simulink model "mrefrobotarm_previous_y_previous_u_previous_ref_cex_3"  (R2018b)
settings: Solver=FixedStepAuto  StartTime=0.0  StopTime=20  RelTol=1e-3  AbsTol=1e-6
undefined symbols (not defined in the file or in its folder): cc, options
libraries: neural x396, simulink x2
(part 9 of 15)

== system mrefrobotarm_previous_y_previous_u_previous_ref_cex_3/cex_m3_adapt/Layer 3/Delays 1 ==
  "p{3}" : Inport  PortDimensions=30
      mask Display: e = 0.06;c1 = [120 230 180]/255;c2 = ([120 230 180]+0)/(256+128);c3 = ([120 230 180]+128)/(256+128);patch([0 1 1 0],[0 0 1 1],c1);patch([0 1 1 1-e 1-e 0+e],[0 0 1 1-e 0+e 0+e],c2);patch([0 0 1 1-e 0+e 0+e],[0 1 1 1-e 1-e 0+e],c3);plot([0 1 1 0 0],[0 0 1 1 0]);
  mux : Mux  Inputs=1
      mask Display: e = 0.06;c1 = [120 150 230]/255;c2 = ([120 150 230]+0)/383;c3 = ([120 150 230]+128)/383;patch([0 1 1 0],[0 0 1 1],c1);patch([0 1 1 1-e 1-e 0+e],[0 0 1 1-e 0+e 0+e],c2);patch([0 0 1 1-e 0+e 0+e],[0 1 1 1-e 1-e 0+e],c3);plot([0 1 1 0 0],[0 0 1 1 0]);disp('Mux')
  "pd{3,2}" : Outport
      mask Display: e = 0.06;c1 = [120 230 180]/255;c2 = ([120 230 180]+0)/(256+128);c3 = ([120 230 180]+128)/(256+128);patch([0 1 1 0],[0 0 1 1],c1);patch([0 1 1 1-e 1-e 0+e],[0 0 1 1-e 0+e 0+e],c2);patch([0 0 1 1-e 0+e 0+e],[0 1 1 1-e 1-e 0+e],c3);plot([0 1 1 0 0],[0 0 1 1 0]);
  wires:
  "p{3}"/1 -> mux/1
  mux/1 -> "pd{3,2}"/1

== system mrefrobotarm_previous_y_previous_u_previous_ref_cex_3/cex_m3_adapt/Layer 3/LW{3,2} ==
  "ad{3,2}" : Inport  PortDimensions=30
      mask Display: e = 0.06;c1 = [120 230 180]/255;c2 = ([120 230 180]+0)/(256+128);c3 = ([120 230 180]+128)/(256+128);patch([0 1 1 0],[0 0 1 1],c1);patch([0 1 1 1-e 1-e 0+e],[0 0 1 1-e 0+e 0+e],c2);patch([0 0 1 1-e 0+e 0+e],[0 1 1 1-e 1-e 0+e],c3);plot([0 1 1 0 0],[0 0 1 1 0]);
  "IW{3,2}(1,:)'" : Constant  Value=[-0.0550595154242625728358007108909077942371368408203125;-0.3289027625891562944815404989640228450298309326171875;0.415393748344756452706150184894795529544353485107421875;-0.2282636721929082457283044504947611130774021148681640625;0.1668741853640021977067675607031560502946376800537109375;-0.287669874496869149016475830649142153561115264892578125;-0.3212911955461403845646373156341724097728729248046875;0.12071215019926258282811915023557958193123340606689453125;-0.0146013532017180598654437773120662313885986804962158203125;0.50163897067026586018556599810835905373096466064453125;0.35771292541943811027493893561768345534801483154296875;-0.00629606603251300737944529117839920218102633953094482421875;-0.04508272836454159382402195888062124140560626983642578125;0.00996937137599121676878599629390009795315563678741455078125;0.285260980440774691846428368080523796379566192626953125;0.2491459745752436505394911137045710347592830657958984375;-0.183824283017604284129475900044781155884265899658203125;0.45987709705359447465156108592054806649684906005859375;0.03695776745205560376295039759497740305960178375244140625;0.038818132468089842912473130809303256683051586151123046875;0.32020077507497279878379004003363661468029022216796875;-0.02219398795991646411440711972318240441381931304931640625;0.176419324787934705955905201335554011166095733642578125;-0.369064045925398043213050414124154485762119293212890625;-0.0296495007456062768802507179088934208266437053680419921875;-0.03653538424870143852540849138677003793418407440185546875;0.278071205950087219083144418618758209049701690673828125;0.5598987685029681582449256893596611917018890380859375;-0.2178278744586039927799703264099662192165851593017578125;0.406415787608162049071580668169190175831317901611328125]
      mask Display: e = 0.06;c1 = [120 150 230]/255;c2 = ([120 150 230]+0)/383;c3 = ([120 150 230]+128)/383;patch([0 1 1 0],[0 0 1 1],c1);patch([0 1 1 1-e 1-e 0+e],[0 0 1 1-e 0+e 0+e],c2);patch([0 0 1 1-e 0+e 0+e],[0 1 1 1-e 1-e 0+e],c3);plot([0 1 1 0 0],[0 0 1 1 0]);disp('weights');
  Mux : Mux  Inputs=1
      mask Display: e = 0.06;c1 = [120 150 230]/255;c2 = ([120 150 230]+0)/383;c3 = ([120 150 230]+128)/383;patch([0 1 1 0],[0 0 1 1],c1);patch([0 1 1 1-e 1-e 0+e],[0 0 1 1-e 0+e 0+e],c2);patch([0 0 1 1-e 0+e 0+e],[0 1 1 1-e 1-e 0+e],c3);plot([0 1 1 0 0],[0 0 1 1 0]);disp('Mux');
  dotprod1 : neural/Weight Functions/dotprod
  "lz{3,2}" : Outport
      mask Display: e = 0.06;c1 = [120 230 180]/255;c2 = ([120 230 180]+0)/(256+128);c3 = ([120 230 180]+128)/(256+128);patch([0 1 1 0],[0 0 1 1],c1);patch([0 1 1 1-e 1-e 0+e],[0 0 1 1-e 0+e 0+e],c2);patch([0 0 1 1-e 0+e 0+e],[0 1 1 1-e 1-e 0+e],c3);plot([0 1 1 0 0],[0 0 1 1 0]);
  wires:
  "IW{3,2}(1,:)'"/1 -> dotprod1/1
  "ad{3,2}"/1 -> dotprod1/2
  dotprod1/1 -> Mux/1
  Mux/1 -> "lz{3,2}"/1

== system mrefrobotarm_previous_y_previous_u_previous_ref_cex_3/cex_m4_10_cl/Layer 1/Delays 1 ==
  "p{1}" : Inport  PortDimensions=10
      mask Display: e = 0.06;c1 = [120 230 180]/255;c2 = ([120 230 180]+0)/(256+128);c3 = ([120 230 180]+128)/(256+128);patch([0 1 1 0],[0 0 1 1],c1);patch([0 1 1 1-e 1-e 0+e],[0 0 1 1-e 0+e 0+e],c2);patch([0 0 1 1-e 0+e 0+e],[0 1 1 1-e 1-e 0+e],c3);plot([0 1 1 0 0],[0 0 1 1 0]);
  mux : Mux  Inputs=1
      mask Display: e = 0.06;c1 = [120 150 230]/255;c2 = ([120 150 230]+0)/383;c3 = ([120 150 230]+128)/383;patch([0 1 1 0],[0 0 1 1],c1);patch([0 1 1 1-e 1-e 0+e],[0 0 1 1-e 0+e 0+e],c2);patch([0 0 1 1-e 0+e 0+e],[0 1 1 1-e 1-e 0+e],c3);plot([0 1 1 0 0],[0 0 1 1 0]);disp('Mux')
  "pd{1,1}" : Outport
      mask Display: e = 0.06;c1 = [120 230 180]/255;c2 = ([120 230 180]+0)/(256+128);c3 = ([120 230 180]+128)/(256+128);patch([0 1 1 0],[0 0 1 1],c1);patch([0 1 1 1-e 1-e 0+e],[0 0 1 1-e 0+e 0+e],c2);patch([0 0 1 1-e 0+e 0+e],[0 1 1 1-e 1-e 0+e],c3);plot([0 1 1 0 0],[0 0 1 1 0]);
  wires:
  "p{1}"/1 -> mux/1
  mux/1 -> "pd{1,1}"/1

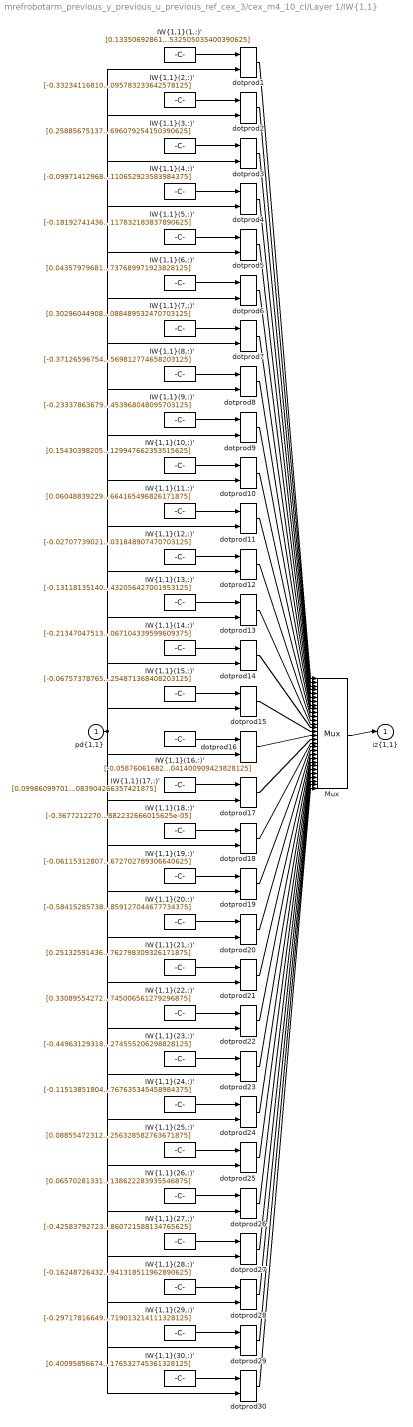
== system mrefrobotarm_previous_y_previous_u_previous_ref_cex_3/cex_m4_10_cl/Layer 1/IW{1,1} ==
  "pd{1,1}" : Inport  PortDimensions=10
      mask Display: e = 0.06;c1 = [120 230 180]/255;c2 = ([120 230 180]+0)/(256+128);c3 = ([120 230 180]+128)/(256+128);patch([0 1 1 0],[0 0 1 1],c1);patch([0 1 1 1-e 1-e 0+e],[0 0 1 1-e 0+e 0+e],c2);patch([0 0 1 1-e 0+e 0+e],[0 1 1 1-e 1-e 0+e],c3);plot([0 1 1 0 0],[0 0 1 1 0]);
  "IW{1,1}(1,:)'" : Constant  Value=[0.1335069286146624290001483359446865506470203399658203125;-0.04119881948015781392147260930869379080832004547119140625;-0.04923129418669790202667257972279912792146205902099609375;-0.11541957449396934853869112203028635121881961822509765625;-0.1293441358240161320747318995927344076335430145263671875;-0.044315180700797374147015261769411154091358184814453125;-0.30838951010690951459736197648453526198863983154296875;0.10507902740775072747414498053331044502556324005126953125;-0.2124968740055101223962452650084742344915866851806640625;0.2253827290816003137141620982220047153532505035400390625]
      mask Display: e = 0.06;c1 = [120 150 230]/255;c2 = ([120 150 230]+0)/383;c3 = ([120 150 230]+128)/383;patch([0 1 1 0],[0 0 1 1],c1);patch([0 1 1 1-e 1-e 0+e],[0 0 1 1-e 0+e 0+e],c2);patch([0 0 1 1-e 0+e 0+e],[0 1 1 1-e 1-e 0+e],c3);plot([0 1 1 0 0],[0 0 1 1 0]);disp('Weights');
  "IW{1,1}(10,:)'" : Constant  Value=[0.1543039820570023257229053115224814973771572113037109375;0.44163458230561747352993506865459494292736053466796875;-0.157209668123826862284886374254710972309112548828125;0.1729117581733836950252936048855190165340900421142578125;0.43717240672936885648169891283032484352588653564453125;-0.185011277685246167123978011659346520900726318359375;0.243474939005600299335441150105907581746578216552734375;-0.0010861071418907385262297982109203076106496155261993408203125;0.1532198832903562124574392555587110109627246856689453125;-0.06418866992842099661320531822639168240129947662353515625]
      mask Display: e = 0.06;c1 = [120 150 230]/255;c2 = ([120 150 230]+0)/383;c3 = ([120 150 230]+128)/383;patch([0 1 1 0],[0 0 1 1],c1);patch([0 1 1 1-e 1-e 0+e],[0 0 1 1-e 0+e 0+e],c2);patch([0 0 1 1-e 0+e 0+e],[0 1 1 1-e 1-e 0+e],c3);plot([0 1 1 0 0],[0 0 1 1 0]);disp('Weights');
  "IW{1,1}(11,:)'" : Constant  Value=[0.0604883922918798833112674628864624537527561187744140625;-0.12877197402082496413555645631277002394199371337890625;-0.0183281447432761500360154371946919127367436885833740234375;-0.17418874047358390289019780539092607796192169189453125;0.0248699482724969618552268713074226980097591876983642578125;0.262836414092244174955936841797665692865848541259765625;-0.134245057446654325605805979648721404373645782470703125;0.1889774580328676123475162285103579051792621612548828125;-0.0915680536010251844292184841833659447729587554931640625;0.074272479267489088794462759324233047664165496826171875]
      mask Display: e = 0.06;c1 = [120 150 230]/255;c2 = ([120 150 230]+0)/383;c3 = ([120 150 230]+128)/383;patch([0 1 1 0],[0 0 1 1],c1);patch([0 1 1 1-e 1-e 0+e],[0 0 1 1-e 0+e 0+e],c2);patch([0 0 1 1-e 0+e 0+e],[0 1 1 1-e 1-e 0+e],c3);plot([0 1 1 0 0],[0 0 1 1 0]);disp('Weights');
  "IW{1,1}(12,:)'" : Constant  Value=[-0.0270773902183627200590532169144353247247636318206787109375;-0.3935532540680071189598265846143476665019989013671875;0.1544558044375887728705265544704161584377288818359375;0.1135619620646874938785231279325671494007110595703125;-0.06923700442986756298235917483907542191445827484130859375;0.023714916382562567509495465856161899864673614501953125;-0.2434424848174343569695565747679211199283599853515625;-0.1940819242046150361336032119652372784912586212158203125;0.1772986216597098041436453286223695613443851470947265625;-0.1902225870534570983938493782261502929031848907470703125]
      mask Display: e = 0.06;c1 = [120 150 230]/255;c2 = ([120 150 230]+0)/383;c3 = ([120 150 230]+128)/383;patch([0 1 1 0],[0 0 1 1],c1);patch([0 1 1 1-e 1-e 0+e],[0 0 1 1-e 0+e 0+e],c2);patch([0 0 1 1-e 0+e 0+e],[0 1 1 1-e 1-e 0+e],c3);plot([0 1 1 0 0],[0 0 1 1 0]);disp('Weights');
  "IW{1,1}(13,:)'" : Constant  Value=[-0.131181351403738821748135023881332017481327056884765625;0.1362970166403306981894871796612278558313846588134765625;-0.0631587600902037415995238234245334751904010772705078125;0.1979319007788440110129357663026894442737102508544921875;-0.14152574162728093210006363733555190265178680419921875;0.00842057206973761095125663445060126832686364650726318359375;0.0918117915633907266670377111950074322521686553955078125;-0.15022518079095015242074850903009064495563507080078125;-0.199192862120646629886522305241669528186321258544921875;0.292466314204549437949509638201561756432056427001953125]
      mask Display: e = 0.06;c1 = [120 150 230]/255;c2 = ([120 150 230]+0)/383;c3 = ([120 150 230]+128)/383;patch([0 1 1 0],[0 0 1 1],c1);patch([0 1 1 1-e 1-e 0+e],[0 0 1 1-e 0+e 0+e],c2);patch([0 0 1 1-e 0+e 0+e],[0 1 1 1-e 1-e 0+e],c3);plot([0 1 1 0 0],[0 0 1 1 0]);disp('Weights');
  "IW{1,1}(14,:)'" : Constant  Value=[-0.21347047513201877766420011539594270288944244384765625;0.016920838378240217469983264209076878614723682403564453125;0.26282359254795928382719694127445109188556671142578125;-0.038626445771948618446156586969664203934371471405029296875;0.01267614658551742719272414916531488415785133838653564453125;0.243713695853148115677555551883415319025516510009765625;0.232007573027820435118684372355346567928791046142578125;0.292359098771159120477847181973629631102085113525390625;-0.1367485882737829727684442104873596690595149993896484375;0.0747256641880101601937980149159557186067104339599609375]
      mask Display: e = 0.06;c1 = [120 150 230]/255;c2 = ([120 150 230]+0)/383;c3 = ([120 150 230]+128)/383;patch([0 1 1 0],[0 0 1 1],c1);patch([0 1 1 1-e 1-e 0+e],[0 0 1 1-e 0+e 0+e],c2);patch([0 0 1 1-e 0+e 0+e],[0 1 1 1-e 1-e 0+e],c3);plot([0 1 1 0 0],[0 0 1 1 0]);disp('Weights');
  "IW{1,1}(15,:)'" : Constant  Value=[-0.067573787655347938851946310023777186870574951171875;-0.295392823875792964738451473749591968953609466552734375;-0.0168225079369467185597120106876900536008179187774658203125;-0.297859471899082295376359752481221221387386322021484375;-0.28145973576240546076832060862216167151927947998046875;-0.2100793210813916844781346071613370440900325775146484375;0.0167045522183084625689186708541456027887761592864990234375;-0.243409163141346918113328001709305681288242340087890625;0.1817946730395441912175868992562755011022090911865234375;-0.018388171280658067996416349387800437398254871368408203125]
      mask Display: e = 0.06;c1 = [120 150 230]/255;c2 = ([120 150 230]+0)/383;c3 = ([120 150 230]+128)/383;patch([0 1 1 0],[0 0 1 1],c1);patch([0 1 1 1-e 1-e 0+e],[0 0 1 1-e 0+e 0+e],c2);patch([0 0 1 1-e 0+e 0+e],[0 1 1 1-e 1-e 0+e],c3);plot([0 1 1 0 0],[0 0 1 1 0]);disp('Weights');
  "IW{1,1}(16,:)'" : Constant  Value=[-0.05876061682829540611106011738229426555335521697998046875;0.360436775341689052964966322178952395915985107421875;0.289705563067306937075073847154271788895130157470703125;0.12081195104620233438108556356382905505597591400146484375;-0.1033261310861984527686985302352695725858211517333984375;0.2466138189248444356760359141844674013555049896240234375;0.21455052857311296410358636421733535826206207275390625;-0.08664495004047449711048756171294371597468852996826171875;0.1862050765935379381676995080852066166698932647705078125;-0.052106136261183162716736916308946092613041400909423828125]
      mask Display: e = 0.06;c1 = [120 150 230]/255;c2 = ([120 150 230]+0)/383;c3 = ([120 150 230]+128)/383;patch([0 1 1 0],[0 0 1 1],c1);patch([0 1 1 1-e 1-e 0+e],[0 0 1 1-e 0+e 0+e],c2);patch([0 0 1 1-e 0+e 0+e],[0 1 1 1-e 1-e 0+e],c3);plot([0 1 1 0 0],[0 0 1 1 0]);disp('Weights');
  "IW{1,1}(17,:)'" : Constant  Value=[0.09986099701258464855779806157443090341985225677490234375;-0.06888901320057617960745943719302886165678501129150390625;-0.09200685624381586824593881601686007343232631683349609375;-0.1891588439145970301780153022264130413532257080078125;0.113842455384469520840440281972405500710010528564453125;0.032373501675791165055340314893328468315303325653076171875;0.0486132218901944579414475811063311994075775146484375;-0.2115118545103817082608799182708025909960269927978515625;-0.2031023047480521592778046624516719020903110504150390625;-0.329202134434376680882650134662981145083904266357421875]
      mask Display: e = 0.06;c1 = [120 150 230]/255;c2 = ([120 150 230]+0)/383;c3 = ([120 150 230]+128)/383;patch([0 1 1 0],[0 0 1 1],c1);patch([0 1 1 1-e 1-e 0+e],[0 0 1 1-e 0+e 0+e],c2);patch([0 0 1 1-e 0+e 0+e],[0 1 1 1-e 1-e 0+e],c3);plot([0 1 1 0 0],[0 0 1 1 0]);disp('Weights');
  "IW{1,1}(18,:)'" : Constant  Value=[-0.3677212270391405635194814749411307275295257568359375;0.05148060778210650223485345122753642499446868896484375;-0.093255280771188997501752737662172876298427581787109375;0.06565608607994800893781217610012390650808811187744140625;-0.225727788425362951851838033690000884234905242919921875;0.09605090868460068598277956652964348904788494110107421875;0.033920970624489343858698475742130540311336517333984375;-0.26114541967138749090082683323998935520648956298828125;0.257344020629603875693902637067367322742938995361328125;-8.736879148670711504875985298212981433607637882232666015625e-05]
      mask Display: e = 0.06;c1 = [120 150 230]/255;c2 = ([120 150 230]+0)/383;c3 = ([120 150 230]+128)/383;patch([0 1 1 0],[0 0 1 1],c1);patch([0 1 1 1-e 1-e 0+e],[0 0 1 1-e 0+e 0+e],c2);patch([0 0 1 1-e 0+e 0+e],[0 1 1 1-e 1-e 0+e],c3);plot([0 1 1 0 0],[0 0 1 1 0]);disp('Weights');
  "IW{1,1}(19,:)'" : Constant  Value=[-0.061153128073666941644237482478274614550173282623291015625;-0.150089827624216354262642880712519399821758270263671875;0.08671999110216542516749171909395954571664333343505859375;-0.0628523003683129355412262384561472572386264801025390625;0.2452322268404465710478490336754475720226764678955078125;-0.10162074530770455471628821442209300585091114044189453125;0.334201538400112851956436088585178367793560028076171875;0.009410034126397896769855577758789877407252788543701171875;-0.1646375700629976457367575903845136053860187530517578125;-0.11189823007734533977242108448990620672702789306640625]
      mask Display: e = 0.06;c1 = [120 150 230]/255;c2 = ([120 150 230]+0)/383;c3 = ([120 150 230]+128)/383;patch([0 1 1 0],[0 0 1 1],c1);patch([0 1 1 1-e 1-e 0+e],[0 0 1 1-e 0+e 0+e],c2);patch([0 0 1 1-e 0+e 0+e],[0 1 1 1-e 1-e 0+e],c3);plot([0 1 1 0 0],[0 0 1 1 0]);disp('Weights');
  "IW{1,1}(2,:)'" : Constant  Value=[-0.3323411681062318212553918783669359982013702392578125;-0.154673593400318776236446183247608132660388946533203125;0.1653441009670726102864790618696133606135845184326171875;0.08240688446507839215460222703768522478640079498291015625;0.286432838047223470301361203382839448750019073486328125;-0.022122764349317834697838947022319189272820949554443359375;-0.00766446205364790418557152662515363772399723529815673828125;-0.1367725418678419069262730545233353041112422943115234375;-0.250579344929661218532856992169399745762348175048828125;0.053861527883418525153302880426053889095783233642578125]
      mask Display: e = 0.06;c1 = [120 150 230]/255;c2 = ([120 150 230]+0)/383;c3 = ([120 150 230]+128)/383;patch([0 1 1 0],[0 0 1 1],c1);patch([0 1 1 1-e 1-e 0+e],[0 0 1 1-e 0+e 0+e],c2);patch([0 0 1 1-e 0+e 0+e],[0 1 1 1-e 1-e 0+e],c3);plot([0 1 1 0 0],[0 0 1 1 0]);disp('Weights');
  "IW{1,1}(20,:)'" : Constant  Value=[-0.58415285738136812909715445130132138729095458984375;0.53930070079611847067013741252594627439975738525390625;-0.197661936388412673437642297358252108097076416015625;-0.1690839785960029095779333374593988992273807525634765625;-0.00690086496233999029115135925849244813434779644012451171875;-0.419685250641533780235903350330772809684276580810546875;-0.09872138899374226228555784246054827235639095306396484375;-0.1627977525170371808638236643673735670745372772216796875;-0.318146809739166924746456288630724884569644927978515625;-0.130148046874022094154810247346176765859127044677734375]
      mask Display: e = 0.06;c1 = [120 150 230]/255;c2 = ([120 150 230]+0)/383;c3 = ([120 150 230]+128)/383;patch([0 1 1 0],[0 0 1 1],c1);patch([0 1 1 1-e 1-e 0+e],[0 0 1 1-e 0+e 0+e],c2);patch([0 0 1 1-e 0+e 0+e],[0 1 1 1-e 1-e 0+e],c3);plot([0 1 1 0 0],[0 0 1 1 0]);disp('Weights');
  "IW{1,1}(21,:)'" : Constant  Value=[0.251325914363370983561907223702291958034038543701171875;0.179997632412586094918793833130621351301670074462890625;0.2489681945741413215955617488361895084381103515625;-0.10037777365444662536209108338880469091236591339111328125;-0.152924777124262278871213993625133298337459564208984375;0.282206938701535847702217552068759687244892120361328125;-0.161723546504821624747449959613732062280178070068359375;0.12769054485279285326981835169135592877864837646484375;0.2150941775257640131702174812744488008320331573486328125;-0.0186245132798998624945596702673356048762798309326171875]
      mask Display: e = 0.06;c1 = [120 150 230]/255;c2 = ([120 150 230]+0)/383;c3 = ([120 150 230]+128)/383;patch([0 1 1 0],[0 0 1 1],c1);patch([0 1 1 1-e 1-e 0+e],[0 0 1 1-e 0+e 0+e],c2);patch([0 0 1 1-e 0+e 0+e],[0 1 1 1-e 1-e 0+e],c3);plot([0 1 1 0 0],[0 0 1 1 0]);disp('Weights');
  "IW{1,1}(22,:)'" : Constant  Value=[0.33089554272644416954562984756194055080413818359375;-0.1924353896389504325892261249464354477822780609130859375;-0.2267754942334463674757927265090984292328357696533203125;-0.0934872108709188243125254302867688238620758056640625;-0.054699933021623577122927173377320286817848682403564453125;0.035072794239530420690176271136806462891399860382080078125;0.26562875685814424375763564967201091349124908447265625;-0.0791922808190812232975730466932873241603374481201171875;0.0521094046242211172970115740099572576582431793212890625;0.339894278826450235708733771389233879745006561279296875]
      mask Display: e = 0.06;c1 = [120 150 230]/255;c2 = ([120 150 230]+0)/383;c3 = ([120 150 230]+128)/383;patch([0 1 1 0],[0 0 1 1],c1);patch([0 1 1 1-e 1-e 0+e],[0 0 1 1-e 0+e 0+e],c2);patch([0 0 1 1-e 0+e 0+e],[0 1 1 1-e 1-e 0+e],c3);plot([0 1 1 0 0],[0 0 1 1 0]);disp('Weights');
  "IW{1,1}(23,:)'" : Constant  Value=[-0.449631293180019764310628715975326485931873321533203125;-0.07520771148848910681028456792773795314133167266845703125;0.201995553128253402253022841250640340149402618408203125;0.0879938416974312687113268793837050907313823699951171875;0.276521095050688614502831796926329843699932098388671875;-0.00327530247935484651600201999599448754452168941497802734375;-0.08464502029784491676789315306450589559972286224365234375;-0.06796671234375029069241236356901936233043670654296875;0.252160726035627058561061630825861357152462005615234375;-0.23821476079948400439434408326633274555206298828125]
      mask Display: e = 0.06;c1 = [120 150 230]/255;c2 = ([120 150 230]+0)/383;c3 = ([120 150 230]+128)/383;patch([0 1 1 0],[0 0 1 1],c1);patch([0 1 1 1-e 1-e 0+e],[0 0 1 1-e 0+e 0+e],c2);patch([0 0 1 1-e 0+e 0+e],[0 1 1 1-e 1-e 0+e],c3);plot([0 1 1 0 0],[0 0 1 1 0]);disp('Weights');
  "IW{1,1}(24,:)'" : Constant  Value=[-0.11513851804525521149713540580705739557743072509765625;0.2108759995406740139767265418413444422185420989990234375;-0.150452927119801349586936112245894037187099456787109375;0.313006723398378483569359786997665651142597198486328125;0.1500465352567468546585160993345198221504688262939453125;0.257667967348261306437251505485619418323040008544921875;0.12369309318535488817492051794033613987267017364501953125;0.07888033237337994940663321585816447623074054718017578125;0.0879306499486552095579128263125312514603137969970703125;0.09146517670438868152782418974311440251767635345458984375]
      mask Display: e = 0.06;c1 = [120 150 230]/255;c2 = ([120 150 230]+0)/383;c3 = ([120 150 230]+128)/383;patch([0 1 1 0],[0 0 1 1],c1);patch([0 1 1 1-e 1-e 0+e],[0 0 1 1-e 0+e 0+e],c2);patch([0 0 1 1-e 0+e 0+e],[0 1 1 1-e 1-e 0+e],c3);plot([0 1 1 0 0],[0 0 1 1 0]);disp('Weights');
  "IW{1,1}(25,:)'" : Constant  Value=[0.0885547231264663670113890248103416524827480316162109375;0.152415072508726268107892565240035764873027801513671875;0.216782935142308896825369401994976215064525604248046875;-0.0011168416512122897495118412081183123518712818622589111328125;-0.1949456192470744031464136014619725756347179412841796875;0.1509795742077182645335398092356626875698566436767578125;-0.0131727055641329589275034805950781446881592273712158203125;0.267350084060445081224344221482169814407825469970703125;0.11563186876736882002791872992020216770470142364501953125;-0.206417403603995353034150639359722845256328582763671875]
      mask Display: e = 0.06;c1 = [120 150 230]/255;c2 = ([120 150 230]+0)/383;c3 = ([120 150 230]+128)/383;patch([0 1 1 0],[0 0 1 1],c1);patch([0 1 1 1-e 1-e 0+e],[0 0 1 1-e 0+e 0+e],c2);patch([0 0 1 1-e 0+e 0+e],[0 1 1 1-e 1-e 0+e],c3);plot([0 1 1 0 0],[0 0 1 1 0]);disp('Weights');
  "IW{1,1}(26,:)'" : Constant  Value=[0.06570281331582818185044203573852428235113620758056640625;0.25845386805039094468838811735622584819793701171875;-0.1705550086578924984248573082368238829076290130615234375;-0.0186638124172070936357403780903041479177772998809814453125;0.1807873632390179230444715585690573789179325103759765625;0.1397273840105673070599578977635246701538562774658203125;0.308961102692036082562054843947407789528369903564453125;0.09885548347453687600960847703390754759311676025390625;-0.0743370873542917587339928786605014465749263763427734375;0.0172194467283331535678581047932311776094138622283935546875]
      mask Display: e = 0.06;c1 = [120 150 230]/255;c2 = ([120 150 230]+0)/383;c3 = ([120 150 230]+128)/383;patch([0 1 1 0],[0 0 1 1],c1);patch([0 1 1 1-e 1-e 0+e],[0 0 1 1-e 0+e 0+e],c2);patch([0 0 1 1-e 0+e 0+e],[0 1 1 1-e 1-e 0+e],c3);plot([0 1 1 0 0],[0 0 1 1 0]);disp('Weights');
  "IW{1,1}(27,:)'" : Constant  Value=[-0.425837927238558788811673139207414351403713226318359375;0.1908390344700196805671765787337790243327617645263671875;-0.07214277970303151210629266643081791698932647705078125;-0.2350904948602744182206691903047612868249416351318359375;-0.039027833323215556371454937334419810213148593902587890625;-0.0601816637202187421085142204901785589754581451416015625;0.18026871997388838053666404448449611663818359375;0.1767672719946612180930145541424280963838100433349609375;0.206184996067080239523505724719143472611904144287109375;-0.03258647382287538363243584171868860721588134765625]
      mask Display: e = 0.06;c1 = [120 150 230]/255;c2 = ([120 150 230]+0)/383;c3 = ([120 150 230]+128)/383;patch([0 1 1 0],[0 0 1 1],c1);patch([0 1 1 1-e 1-e 0+e],[0 0 1 1-e 0+e 0+e],c2);patch([0 0 1 1-e 0+e 0+e],[0 1 1 1-e 1-e 0+e],c3);plot([0 1 1 0 0],[0 0 1 1 0]);disp('Weights');
  "IW{1,1}(28,:)'" : Constant  Value=[-0.1624872643289380358400109116701059974730014801025390625;0.03594315329252119328717895996305742301046848297119140625;0.142750905908062775129252486294717527925968170166015625;-0.01589910599028530879817111554075381718575954437255859375;0.148499745419180040340023651879164390265941619873046875;-0.18266582034752010255118648274219594895839691162109375;-0.1182097013082769876302080547247896902263164520263671875;0.128590777238574760499290050574927590787410736083984375;0.19889063255425643017559877989697270095348358154296875;0.001203452995617513600346004665198051952756941318511962890625]
      mask Display: e = 0.06;c1 = [120 150 230]/255;c2 = ([120 150 230]+0)/383;c3 = ([120 150 230]+128)/383;patch([0 1 1 0],[0 0 1 1],c1);patch([0 1 1 1-e 1-e 0+e],[0 0 1 1-e 0+e 0+e],c2);patch([0 0 1 1-e 0+e 0+e],[0 1 1 1-e 1-e 0+e],c3);plot([0 1 1 0 0],[0 0 1 1 0]);disp('Weights');
  "IW{1,1}(29,:)'" : Constant  Value=[-0.297178166492661599562552510178647935390472412109375;-0.10126684500560804991220464899015496484935283660888671875;0.035227495004671212364133481287353788502514362335205078125;-0.22314089963038863384525711808237247169017791748046875;0.1267187649834307372476160935548250563442707061767578125;-0.1699139905648407722349446657972293905913829803466796875;-0.10882719121949273322069728919814224354922771453857421875;-0.243246901839678175694103856585570611059665679931640625;-0.197486433416583506694763627820066176354885101318359375;0.1380023506128389698677239039170672185719013214111328125]
      mask Display: e = 0.06;c1 = [120 150 230]/255;c2 = ([120 150 230]+0)/383;c3 = ([120 150 230]+128)/383;patch([0 1 1 0],[0 0 1 1],c1);patch([0 1 1 1-e 1-e 0+e],[0 0 1 1-e 0+e 0+e],c2);patch([0 0 1 1-e 0+e 0+e],[0 1 1 1-e 1-e 0+e],c3);plot([0 1 1 0 0],[0 0 1 1 0]);disp('Weights');
  "IW{1,1}(3,:)'" : Constant  Value=[0.25885675137338604034908939865999855101108551025390625;0.272199459665050491619098238516016863286495208740234375;0.220635260260065191317835342488251626491546630859375;0.28943358387100293072080603451468050479888916015625;0.311519070189319513541903461373294703662395477294921875;0.159647036695979849252324811459402553737163543701171875;0.14291110551886732071835695023764856159687042236328125;0.16899843830983585224458920492907054722309112548828125;0.1566153932913868229714893232085159979760646820068359375;0.0219481309776807000100351530136322253383696079254150390625]
      mask Display: e = 0.06;c1 = [120 150 230]/255;c2 = ([120 150 230]+0)/383;c3 = ([120 150 230]+128)/383;patch([0 1 1 0],[0 0 1 1],c1);patch([0 1 1 1-e 1-e 0+e],[0 0 1 1-e 0+e 0+e],c2);patch([0 0 1 1-e 0+e 0+e],[0 1 1 1-e 1-e 0+e],c3);plot([0 1 1 0 0],[0 0 1 1 0]);disp('Weights');
  "IW{1,1}(30,:)'" : Constant  Value=[0.40095856674866936497636515923659317195415496826171875;0.1267807278977244322959450073540210723876953125;-0.065760640049687679731249545511673204600811004638671875;0.2340706377952722350155312369679450057446956634521484375;0.007897112111206312790034900217506219632923603057861328125;-0.178846342738135544170319235490751452744007110595703125;-0.07638342050952738604419067769413231872022151947021484375;-0.1566868906521251270103078923057182691991329193115234375;0.07813752023629098875101561816336470656096935272216796875;0.30613880183392883083115521003492176532745361328125]
      mask Display: e = 0.06;c1 = [120 150 230]/255;c2 = ([120 150 230]+0)/383;c3 = ([120 150 230]+128)/383;patch([0 1 1 0],[0 0 1 1],c1);patch([0 1 1 1-e 1-e 0+e],[0 0 1 1-e 0+e 0+e],c2);patch([0 0 1 1-e 0+e 0+e],[0 1 1 1-e 1-e 0+e],c3);plot([0 1 1 0 0],[0 0 1 1 0]);disp('Weights');
  "IW{1,1}(4,:)'" : Constant  Value=[-0.09971412968880087601686312837045988999307155609130859375;-0.389186881596281952777616197636234574019908905029296875;0.156560399350727019740503465072833932936191558837890625;-0.0721831557508139931567114899735315702855587005615234375;0.03533190691612399236820607484332867898046970367431640625;0.165812409755197676108906534864217974245548248291015625;-0.0192806554428879284301956431590951979160308837890625;-0.07336077149727736335105277021284564398229122161865234375;-0.5374331887406491592429347292636521160602569580078125;0.095214447510887312287053418913274072110652923583984375]
      mask Display: e = 0.06;c1 = [120 150 230]/255;c2 = ([120 150 230]+0)/383;c3 = ([120 150 230]+128)/383;patch([0 1 1 0],[0 0 1 1],c1);patch([0 1 1 1-e 1-e 0+e],[0 0 1 1-e 0+e 0+e],c2);patch([0 0 1 1-e 0+e 0+e],[0 1 1 1-e 1-e 0+e],c3);plot([0 1 1 0 0],[0 0 1 1 0]);disp('Weights');
  "IW{1,1}(5,:)'" : Constant  Value=[-0.1819274143655069952973946101337787695229053497314453125;-0.2013165411018340289484029881350579671561717987060546875;-0.095600498291309732312726055170060135424137115478515625;0.045409133269961772516598585980318603105843067169189453125;-0.041299648836076292834906809048334253020584583282470703125;0.066479243806390198034961258599651046097278594970703125;-0.1723865937260496694616307422620593570172786712646484375;-0.209451693132997107671400272010941989719867706298828125;0.178651168512874491955955136290867812931537628173828125;-0.11773786843471302498986830187277519144117832183837890625]
      mask Display: e = 0.06;c1 = [120 150 230]/255;c2 = ([120 150 230]+0)/383;c3 = ([120 150 230]+128)/383;patch([0 1 1 0],[0 0 1 1],c1);patch([0 1 1 1-e 1-e 0+e],[0 0 1 1-e 0+e 0+e],c2);patch([0 0 1 1-e 0+e 0+e],[0 1 1 1-e 1-e 0+e],c3);plot([0 1 1 0 0],[0 0 1 1 0]);disp('Weights');
  "IW{1,1}(6,:)'" : Constant  Value=[0.043579796816272380055590218717043171636760234832763671875;0.06504685486043419728741099561375449411571025848388671875;0.101820639984425920232524731545709073543548583984375;-0.1812565686033276446398332382159424014389514923095703125;0.1608154968478545943089130787484464235603809356689453125;-0.136009446913428255765410312960739247500896453857421875;-0.21859454992482307833512322758906520903110504150390625;-0.0406754494486426254606925567713915370404720306396484375;-0.11534446906559632506361623427437734790146350860595703125;0.09306812129286252954774028012252529151737689971923828125]
      mask Display: e = 0.06;c1 = [120 150 230]/255;c2 = ([120 150 230]+0)/383;c3 = ([120 150 230]+128)/383;patch([0 1 1 0],[0 0 1 1],c1);patch([0 1 1 1-e 1-e 0+e],[0 0 1 1-e 0+e 0+e],c2);patch([0 0 1 1-e 0+e 0+e],[0 1 1 1-e 1-e 0+e],c3);plot([0 1 1 0 0],[0 0 1 1 0]);disp('Weights');
  "IW{1,1}(7,:)'" : Constant  Value=[0.3029604490883477385665401016012765467166900634765625;-0.153428082480172423007758197854855097830295562744140625;0.294956104261068274841051106704981066286563873291015625;0.282458371819714171291337834190926514565944671630859375;0.07793099196308429787993787840605364181101322174072265625;0.13330806760957980561244085038197226822376251220703125;0.16836043990242954837555089397937990725040435791015625;0.281483329751889665981678945172461681067943572998046875;-0.0137999067128776464752348829279071651399135589599609375;0.343715411062013143084215016642701812088489532470703125]
      mask Display: e = 0.06;c1 = [120 150 230]/255;c2 = ([120 150 230]+0)/383;c3 = ([120 150 230]+128)/383;patch([0 1 1 0],[0 0 1 1],c1);patch([0 1 1 1-e 1-e 0+e],[0 0 1 1-e 0+e 0+e],c2);patch([0 0 1 1-e 0+e 0+e],[0 1 1 1-e 1-e 0+e],c3);plot([0 1 1 0 0],[0 0 1 1 0]);disp('Weights');
  "IW{1,1}(8,:)'" : Constant  Value=[-0.371265967540699681759264194624847732484340667724609375;-0.06692634591494457663163331062605720944702625274658203125;-0.278459704997866375197901334104244597256183624267578125;-0.23710345870841831317221704011899419128894805908203125;0.044465858191620834249935256821117945946753025054931640625;-0.1994083467870570725022361102674040012061595916748046875;0.1276517852930483254425553241162560880184173583984375;0.1496476237377059315125649163746857084333896636962890625;-0.07075665307495183908859104349176050163805484771728515625;-0.08656163720639516168109395266583305783569812774658203125]
      mask Display: e = 0.06;c1 = [120 150 230]/255;c2 = ([120 150 230]+0)/383;c3 = ([120 150 230]+128)/383;patch([0 1 1 0],[0 0 1 1],c1);patch([0 1 1 1-e 1-e 0+e],[0 0 1 1-e 0+e 0+e],c2);patch([0 0 1 1-e 0+e 0+e],[0 1 1 1-e 1-e 0+e],c3);plot([0 1 1 0 0],[0 0 1 1 0]);disp('Weights');
  "IW{1,1}(9,:)'" : Constant  Value=[-0.233378636799206284901941899079247377812862396240234375;-0.15354110887183025635494004745851270854473114013671875;-0.0263068694725183231664100702573705348186194896697998046875;0.087592869030917286377047048517852090299129486083984375;0.05368505550786541180574573672856786288321018218994140625;-0.037760079152627523679797150180093012750148773193359375;-0.270248117562853218398544186129583977162837982177734375;0.338965049902449300223139516674564220011234283447265625;0.05207849597805429275876321071336860768496990203857421875;-0.01545517607820139256713520836683528614230453968048095703125]
      mask Display: e = 0.06;c1 = [120 150 230]/255;c2 = ([120 150 230]+0)/383;c3 = ([120 150 230]+128)/383;patch([0 1 1 0],[0 0 1 1],c1);patch([0 1 1 1-e 1-e 0+e],[0 0 1 1-e 0+e 0+e],c2);patch([0 0 1 1-e 0+e 0+e],[0 1 1 1-e 1-e 0+e],c3);plot([0 1 1 0 0],[0 0 1 1 0]);disp('Weights');
  Mux : Mux  Inputs=30
      mask Display: e = 0.06;c1 = [120 150 230]/255;c2 = ([120 150 230]+0)/383;c3 = ([120 150 230]+128)/383;patch([0 1 1 0],[0 0 1 1],c1);patch([0 1 1 1-e 1-e 0+e],[0 0 1 1-e 0+e 0+e],c2);patch([0 0 1 1-e 0+e 0+e],[0 1 1 1-e 1-e 0+e],c3);plot([0 1 1 0 0],[0 0 1 1 0]);disp('Mux');
  dotprod{1..30} (30 alike) : neural/Weight Functions/dotprod
  "iz{1,1}" : Outport
      mask Display: e = 0.06;c1 = [120 230 180]/255;c2 = ([120 230 180]+0)/(256+128);c3 = ([120 230 180]+128)/(256+128);patch([0 1 1 0],[0 0 1 1],c1);patch([0 1 1 1-e 1-e 0+e],[0 0 1 1-e 0+e 0+e],c2);patch([0 0 1 1-e 0+e 0+e],[0 1 1 1-e 1-e 0+e],c3);plot([0 1 1 0 0],[0 0 1 1 0]);
  wires:
  "IW{1,1}(1,:)'"/1 -> dotprod1/1
  "pd{1,1}"/1 -> dotprod1/2, dotprod2/2, dotprod3/2, dotprod4/2, dotprod5/2, dotprod6/2, dotprod7/2, dotprod8/2, dotprod9/2, dotprod10/2, dotprod11/2, dotprod12/2, dotprod13/2, dotprod14/2, dotprod15/2, dotprod16/2, dotprod17/2, dotprod18/2, dotprod19/2, dotprod20/2, dotprod21/2, dotprod22/2, dotprod23/2, dotprod24/2, dotprod25/2, dotprod26/2, dotprod27/2, dotprod28/2, dotprod29/2, dotprod30/2
  dotprod1/1 -> Mux/1
  "IW{1,1}(2,:)'"/1 -> dotprod2/1
  dotprod2/1 -> Mux/2
  "IW{1,1}(3,:)'"/1 -> dotprod3/1
  dotprod3/1 -> Mux/3
  "IW{1,1}(4,:)'"/1 -> dotprod4/1
  dotprod4/1 -> Mux/4
  "IW{1,1}(5,:)'"/1 -> dotprod5/1
  dotprod5/1 -> Mux/5
  "IW{1,1}(6,:)'"/1 -> dotprod6/1
  dotprod6/1 -> Mux/6
  "IW{1,1}(7,:)'"/1 -> dotprod7/1
  dotprod7/1 -> Mux/7
  "IW{1,1}(8,:)'"/1 -> dotprod8/1
  dotprod8/1 -> Mux/8
  "IW{1,1}(9,:)'"/1 -> dotprod9/1
  dotprod9/1 -> Mux/9
  "IW{1,1}(10,:)'"/1 -> dotprod10/1
  dotprod10/1 -> Mux/10
  "IW{1,1}(11,:)'"/1 -> dotprod11/1
  dotprod11/1 -> Mux/11
  "IW{1,1}(12,:)'"/1 -> dotprod12/1
  dotprod12/1 -> Mux/12
  "IW{1,1}(13,:)'"/1 -> dotprod13/1
  dotprod13/1 -> Mux/13
  "IW{1,1}(14,:)'"/1 -> dotprod14/1
  dotprod14/1 -> Mux/14
  "IW{1,1}(15,:)'"/1 -> dotprod15/1
  dotprod15/1 -> Mux/15
  "IW{1,1}(16,:)'"/1 -> dotprod16/1
  dotprod16/1 -> Mux/16
  "IW{1,1}(17,:)'"/1 -> dotprod17/1
  dotprod17/1 -> Mux/17
  "IW{1,1}(18,:)'"/1 -> dotprod18/1
  dotprod18/1 -> Mux/18
  "IW{1,1}(19,:)'"/1 -> dotprod19/1
  dotprod19/1 -> Mux/19
  "IW{1,1}(20,:)'"/1 -> dotprod20/1
  dotprod20/1 -> Mux/20
  "IW{1,1}(21,:)'"/1 -> dotprod21/1
  dotprod21/1 -> Mux/21
  "IW{1,1}(22,:)'"/1 -> dotprod22/1
  dotprod22/1 -> Mux/22
  "IW{1,1}(23,:)'"/1 -> dotprod23/1
  dotprod23/1 -> Mux/23
  "IW{1,1}(24,:)'"/1 -> dotprod24/1
  dotprod24/1 -> Mux/24
  "IW{1,1}(25,:)'"/1 -> dotprod25/1
  dotprod25/1 -> Mux/25
  "IW{1,1}(26,:)'"/1 -> dotprod26/1
  dotprod26/1 -> Mux/26
  "IW{1,1}(27,:)'"/1 -> dotprod27/1
  dotprod27/1 -> Mux/27
  "IW{1,1}(28,:)'"/1 -> dotprod28/1
  dotprod28/1 -> Mux/28
  "IW{1,1}(29,:)'"/1 -> dotprod29/1
  dotprod29/1 -> Mux/29
  "IW{1,1}(30,:)'"/1 -> dotprod30/1
  dotprod30/1 -> Mux/30
  Mux/1 -> "iz{1,1}"/1

== system mrefrobotarm_previous_y_previous_u_previous_ref_cex_3/cex_m4_10_cl/Layer 2/Delays 1 ==
  "p{2}" : Inport  PortDimensions=30
      mask Display: e = 0.06;c1 = [120 230 180]/255;c2 = ([120 230 180]+0)/(256+128);c3 = ([120 230 180]+128)/(256+128);patch([0 1 1 0],[0 0 1 1],c1);patch([0 1 1 1-e 1-e 0+e],[0 0 1 1-e 0+e 0+e],c2);patch([0 0 1 1-e 0+e 0+e],[0 1 1 1-e 1-e 0+e],c3);plot([0 1 1 0 0],[0 0 1 1 0]);
  mux : Mux  Inputs=1
      mask Display: e = 0.06;c1 = [120 150 230]/255;c2 = ([120 150 230]+0)/383;c3 = ([120 150 230]+128)/383;patch([0 1 1 0],[0 0 1 1],c1);patch([0 1 1 1-e 1-e 0+e],[0 0 1 1-e 0+e 0+e],c2);patch([0 0 1 1-e 0+e 0+e],[0 1 1 1-e 1-e 0+e],c3);plot([0 1 1 0 0],[0 0 1 1 0]);disp('Mux')
  "pd{2,1}" : Outport
      mask Display: e = 0.06;c1 = [120 230 180]/255;c2 = ([120 230 180]+0)/(256+128);c3 = ([120 230 180]+128)/(256+128);patch([0 1 1 0],[0 0 1 1],c1);patch([0 1 1 1-e 1-e 0+e],[0 0 1 1-e 0+e 0+e],c2);patch([0 0 1 1-e 0+e 0+e],[0 1 1 1-e 1-e 0+e],c3);plot([0 1 1 0 0],[0 0 1 1 0]);
  wires:
  "p{2}"/1 -> mux/1
  mux/1 -> "pd{2,1}"/1
